simulink model "exp_template"  (R2024a)
settings: Solver=FixedStepAuto  StartTime=0.0  StopTime=inf  FixedStep=Ts  RelTol=1e-3
InitFcn:
  | setup
values from neighbouring files (symbols this model uses):
  Ts_Rec = 0.5e-3    (= 0.0005)    [setup.m]
  Ts_Send = 0.5e-3    (= 0.0005)    [setup.m]
undefined symbols (not defined in the file or in its folder): Serial_Port, Standard_Devices
libraries: sldrtlib x4
settings Model: SimulationMode=external  Creator=erman  LastModifiedBy=DBCHNPC
settings HardwareCC: ProdBitPerLong=64  ProdHWDeviceType=Intel->x86-64 (Linux 64)
settings RTWCC: Description=Simulink Desktop Real-Time  SystemTargetFile=sldrt.tlc  TemplateMakefile=sldrt.tmf  RTWCompilerOptimization=on  GPUComputeCapability=3.5
settings CodeAppCC: MaxIdLength=95
settings SimulinkDesktopRealTimeCC: TargetLibSuffix=_sldrt.a  TargetPreCompLibLocation=C:\Program Files\MATLAB\R2024a\toolbox\sldrt\lib\win64

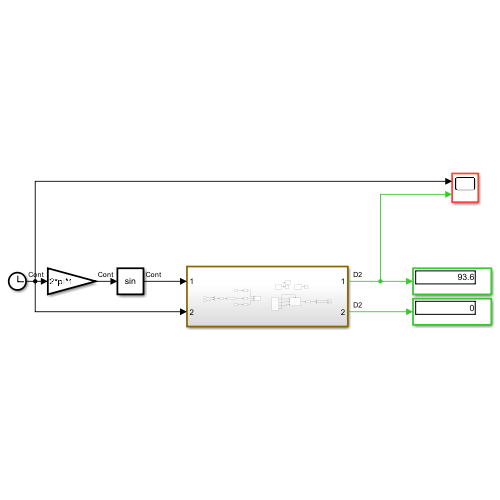
[thumbnail: Simulink's stored preview of the top-level diagram]
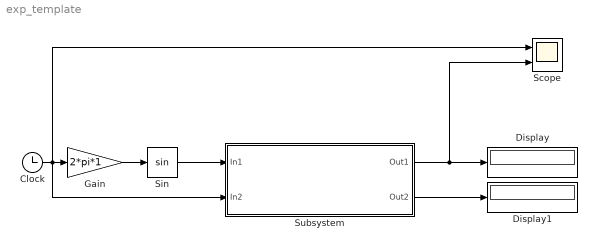
== system exp_template ==
  Clock : Clock
  Display : Display
  Display1 : Display
  Gain : Gain  Gain=2*pi*1
  Scope : Scope  NumInputPorts=2
  Sin : Trigonometry
  Subsystem : Subsystem
  wires:
  Subsystem/1(Out1) -> Scope/2, Display/1
  Sin/1 -> Subsystem/1(In1)
  Clock/1 -> Subsystem/2(In2), Scope/1, Gain/1
  Gain/1 -> Sin/1
  Subsystem/2(Out2) -> Display1/1

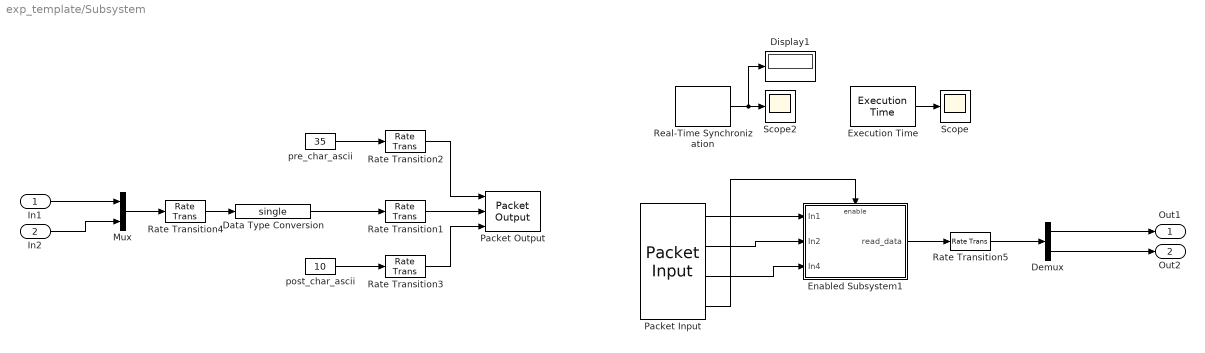
== system exp_template/Subsystem ==
  In1 : Inport
  In2 : Inport  Port=2
  Data Type Conversion : DataTypeConversion  OutDataTypeStr=single  SaturateOnIntegerOverflow=off  RndMeth=Floor
  Demux : Demux  Outputs=2
  Display1 : Display
  Enabled Subsystem1 : Subsystem  TreatAsAtomicUnit=on
  Execution Time : sldrtlib/Target Profiling/Execution Time  ShowTaskTimes=off
  Mux : Mux  Inputs=2
  Packet Input : sldrtlib/Packet Input  SampleTime=Ts_Rec  MaxMissedTicks=1000  ShowMissedTicks=off  YieldWhenWaiting=off  DrvName=Standard_Devices/Serial_Port  DrvAddress=4  DrvOptions=[9600 8 0 0 0 0 0 0]  PacketSize=10  DataTypes={'int8','2*single','int8'}  ShowReady=on  ShowError=off  PacketID=1  ByteOrder=1  ShowTimestamp=off
      settings: AttributesFormatString=Serial Port [4]
  Packet Output : sldrtlib/Packet Output  SampleTime=Ts_Send  MaxMissedTicks=1000  ShowMissedTicks=off  YieldWhenWaiting=off  DrvName=Standard_Devices/Serial_Port  DrvAddress=4  DrvOptions=[9600 8 0 0 0 0 0 0]  PacketSize=10  DataTypes={'int8','2*single','int8'}  ShowReady=off  ShowError=off  PacketID=1  ByteOrder=1  InitialValue=[]  FinalValue=[]
      settings: AttributesFormatString=Serial Port [4]
  Rate Transition1 : RateTransition
  Rate Transition2 : RateTransition
  Rate Transition3 : RateTransition
  Rate Transition4 : RateTransition  OutPortSampleTime=Ts_Send
  Rate Transition5 : RateTransition  OutPortSampleTime=Ts_Algo
  Real-Time Synchronization : sldrtlib/Real-Time Synchronization  SampleTime=Ts_Rec  MaxMissedTicks=1000  ShowMissedTicks=on  YieldWhenWaiting=off
  Scope : Scope
  Scope2 : Scope
  post_char_ascii : Constant  Value=10  OutDataTypeStr=int8  SampleTime=-1
  pre_char_ascii : Constant  Value=35  OutDataTypeStr=int8  SampleTime=-1
  Out1 : Outport
  Out2 : Outport  Port=2
  wires:
  Rate Transition2/1 -> Packet Output/1
  Data Type Conversion/1 -> Rate Transition1/1
  post_char_ascii/1 -> Rate Transition3/1
  In1/1 -> Mux/1
  Packet Input/1 -> Enabled Subsystem1/1(In1)
  Packet Input/2 -> Enabled Subsystem1/2(In2)
  Enabled Subsystem1/1(read_data) -> Rate Transition5/1
  Rate Transition1/1 -> Packet Output/2
  Packet Input/3 -> Enabled Subsystem1/3(In4)
  Execution Time/1 -> Scope/1
  Real-Time Synchronization/1 -> Scope2/1, Display1/1
  pre_char_ascii/1 -> Rate Transition2/1
  Packet Input/4 -> Enabled Subsystem1/Enable
  Rate Transition3/1 -> Packet Output/3
  Rate Transition4/1 -> Data Type Conversion/1
  Mux/1 -> Rate Transition4/1
  In2/1 -> Mux/2
  Rate Transition5/1 -> Demux/1
  Demux/2 -> Out2/1
  Demux/1 -> Out1/1

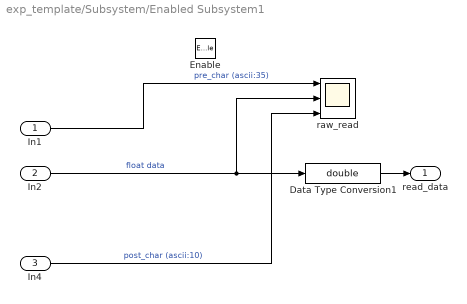
== system exp_template/Subsystem/Enabled Subsystem1 ==
  In1 : Inport
  In2 : Inport  Port=2
  In4 : Inport  Port=3
  Enable : EnablePort
  Data Type Conversion1 : DataTypeConversion  OutDataTypeStr=double  SaturateOnIntegerOverflow=off  RndMeth=Floor
  raw_read : Scope  NumInputPorts=3
  read_data : Outport
  wires:
  Data Type Conversion1/1 -> read_data/1
  In4/1 -> raw_read/3  "post_char (ascii:10)"
  In2/1 -> raw_read/2, Data Type Conversion1/1  "float data"
  In1/1 -> raw_read/1  "pre_char (ascii:35)"
